simulink model "Speed Control"  (R2023a)
settings: Solver=VariableStepAuto  StartTime=0.0  StopTime=10.0  RelTol=1e-3
undefined symbols (not defined in the file or in its folder): L, R
settings Model: Creator=Sadiq Ali  LastModifiedBy=Sadiq Ali

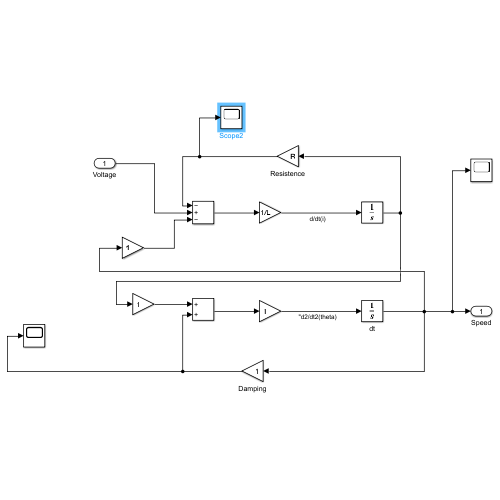
[thumbnail: Simulink's stored preview of the top-level diagram]
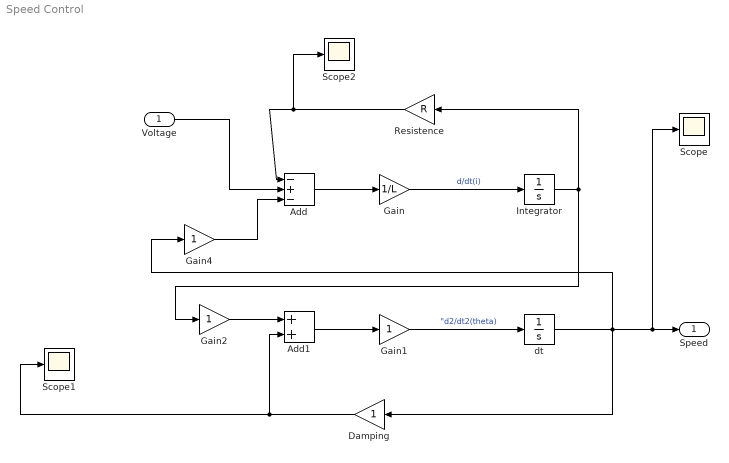
== system Speed Control ==
  Voltage : Inport
  Add : Sum  Inputs=-+-
  Add1 : Sum
  Damping : Gain
  Gain : Gain  Gain=1/L
  Gain1 : Gain
  Gain2 : Gain
  Gain4 : Gain
  Integrator : Integrator
  Resistence : Gain  Gain=R
  Scope : Scope
  Scope1 : Scope
  Scope2 : Scope
  dt : Integrator
  Speed : Outport
  wires:
  Gain/1 -> Integrator/1  "d/dt(i)"
  Gain1/1 -> dt/1  "\"d2/dt2(theta)"
  Add/1 -> Gain/1
  Add1/1 -> Gain1/1
  Gain2/1 -> Add1/1
  Integrator/1 -> Gain2/1, Resistence/1
  Voltage/1 -> Add/2
  Gain4/1 -> Add/3
  Resistence/1 -> Scope2/1, Add/1
  dt/1 -> Scope/1, Speed/1, Damping/1, Gain4/1
  Damping/1 -> Scope1/1, Add1/2
